simulink model "ee5101_3"  (R2023b)
settings: Solver=VariableStepAuto  StartTime=0.0  StopTime=10.0  RelTol=1e-3
values from neighbouring files (symbols this model uses):
  A = [-8.8487+(a-b)/5  -0.0399  -5.5500+(c+d)/10   3.5846 ... (first row only)    [ee5101_1.m]    (also in ee5101_2.m; ee5101_3.m; ee5101_5.m; ee5103_4.m)
  B = [0.0564+(b/(10+c)) ,0.0319 ... (first row only)    [ee5101_1.m]    (also in ee5101_2.m; ee5101_3.m; ee5101_5.m; ee5103_4.m)
  C = [-3.2988, -2.1932+(10*c +d)/(100+5*a) ,0.0370 ,-0.0109 ... (first row only)    [ee5101_1.m]    (also in ee5101_2.m; ee5101_3.m; ee5101_5.m; ee5103_4.m)
  K = Kbar *T    [ee5101_1.m]    (also in ee5101_2.m = real(a*P); ee5101_3.m = a*P; ee5103_4.m = F*C_ss)
  L = K_'    [ee5101_3.m]
settings Model: Creator=perrymiao  LastModifiedBy=perrymiao

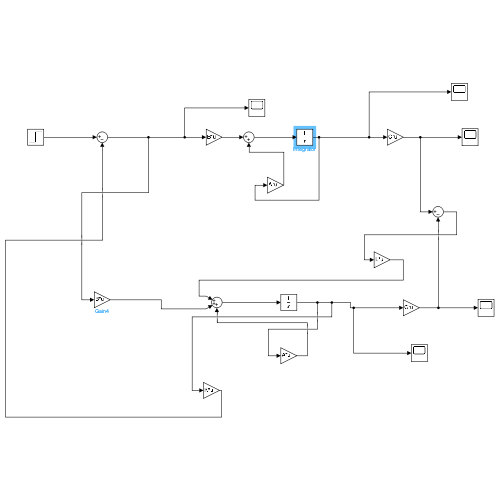
[thumbnail: Simulink's stored preview of the top-level diagram]
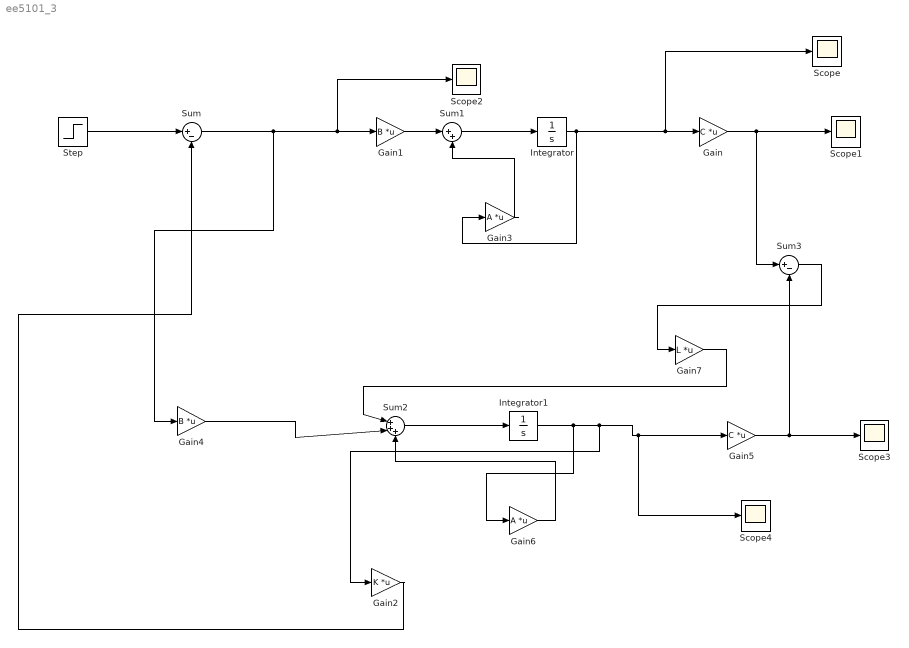
== system ee5101_3 ==
  Gain : Gain  Gain=C  Multiplication=Matrix(K*u)
  Gain1 : Gain  Gain=B  Multiplication=Matrix(K*u)
  Gain2 : Gain  Gain=K  Multiplication=Matrix(K*u)
  Gain3 : Gain  Gain=A  Multiplication=Matrix(K*u)
  Gain4 : Gain  Gain=B  Multiplication=Matrix(K*u)
  Gain5 : Gain  Gain=C  Multiplication=Matrix(K*u)
  Gain6 : Gain  Gain=A  Multiplication=Matrix(K*u)
  Gain7 : Gain  Gain=L  Multiplication=Matrix(K*u)
  Integrator : Integrator
  Integrator1 : Integrator
  Scope{,1..4} (5 alike) : Scope
  Step : Step  Time=0  Before=[0 0]  After=[0 1]  SampleTime=0
  Sum : Sum  Inputs=|+-
  Sum1 : Sum  Inputs=|++
  Sum2 : Sum  Inputs=|+++
  Sum3 : Sum  Inputs=|+-
  wires:
  Sum1/1 -> Integrator/1
  Gain3/1 -> Sum1/2
  Gain/1 -> Scope1/1, Sum3/1
  Sum/1 -> Gain4/1, Scope2/1, Gain1/1
  Gain1/1 -> Sum1/1
  Step/1 -> Sum/1
  Integrator/1 -> Gain3/1, Scope/1, Gain/1
  Gain4/1 -> Sum2/2
  Sum2/1 -> Integrator1/1
  Integrator1/1 -> Gain6/1, Gain2/1, Gain5/1, Scope4/1
  Gain6/1 -> Sum2/3
  Gain5/1 -> Scope3/1, Sum3/2
  Sum3/1 -> Gain7/1
  Gain7/1 -> Sum2/1
  Gain2/1 -> Sum/2
